simulink model "FIRB"  (R2020a)
settings: Solver=VariableStepAuto  StartTime=0.0  StopTime=300  RelTol=1e-3
InitFcn:
  | variableCalc
values from neighbouring files (symbols this model uses):
  aD1 = 10    [variableCalc.m]
  aD2 = 1    [variableCalc.m]
  Alin = [(-1),0,0,0;1,0,0,0;(-1),0,0,0.981E1;0,0,1,0]    [Matrix.m]
  bd = zeros(3,1)    [variableCalc.m]
  Blin = [1;0;1;0]    [Matrix.m]
  cAll = eye(length(Alin))    [variableCalc.m]
  cd = eye(3)    [variableCalc.m]
  d0 = [aD1;0;aD2]    [variableCalc.m]
  dAll = zeros(length(Alin),1)    [variableCalc.m]
  dd = zeros(3,1)    [variableCalc.m]
  S = [0 0 0 ... (first row only)    [variableCalc.m]
  wD1 = 10    [variableCalc.m]
  wD2 = 0.1    [variableCalc.m]
  x0 = [0;1;0;1]    [variableCalc.m]
settings Model: Creator=alfystar  LastModifiedBy=alfystar

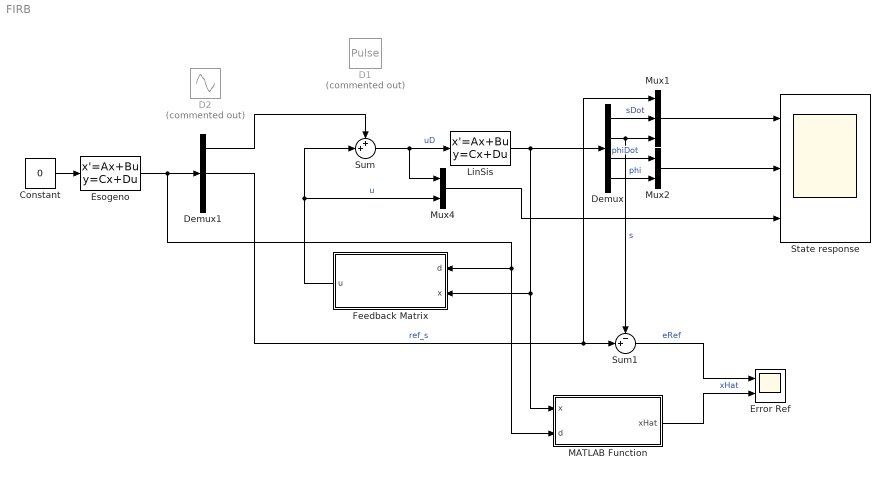
== system FIRB ==
  Constant : Constant  Value=0
  D1 : DiscretePulseGenerator  Commented=on  PulseType=Time based  Amplitude=aD1  Period=wD1  PulseWidth=50
  D2 : Sin  Commented=on  Amplitude=aD2  Frequency=wD2  SampleTime=0
  Demux : Demux
  Demux1 : Demux  Outputs=3
  Error Ref : Scope  NumInputPorts=2
  Esogeno : StateSpace  A=S  B=bd  C=cd  D=dd  InitialCondition=d0
  Feedback Matrix : MATLAB Function  TreatAsAtomicUnit=on
  LinSis : StateSpace  A=Alin  B=Blin  C=cAll  D=dAll  InitialCondition=x0
  MATLAB Function : MATLAB Function  TreatAsAtomicUnit=on
  Mux1 : Mux  Inputs=3
  Mux2 : Mux  Inputs=2
  Mux4 : Mux  Inputs=2
  State response : Scope  NumInputPorts=3
  Sum : Sum  Inputs=++|
  Sum1 : Sum  Inputs=-+|
  wires:
  LinSis/1 -> MATLAB Function/1(x), Feedback Matrix/2(x), Demux/1
  Demux/3 -> Mux2/1  "phiDot"
  Demux/4 -> Mux2/2  "phi"
  Mux1/1 -> State response/1
  Feedback Matrix/1(u) -> Sum/2, Mux4/2  "u"
  Demux/1 -> Mux1/2  "sDot"
  Demux/2 -> Mux1/3, Sum1/1  "s"
  Demux1/2 -> Sum1/2, Mux1/1  "ref_s"
  Mux2/1 -> State response/2
  Sum/1 -> Mux4/1, LinSis/1  "uD"
  Esogeno/1 -> Demux1/1, MATLAB Function/2(d), Feedback Matrix/1(d)
  Constant/1 -> Esogeno/1
  Mux4/1 -> State response/3
  Demux1/1 -> Sum/1
  Sum1/1 -> Error Ref/1  "eRef"
  MATLAB Function/1(xHat) -> Error Ref/2  "xHat"

== matlab function FIRB/MATLAB Function ==
  data: x input; xHat output; d input
function xHat = baseChange(x,d)

coder.extrinsic('evalin', 'assignin')
PiMat = zeros(4,3);                  % Needed in order to set variable class correctly
PiMat = evalin('base','PiMat'); % Read value from workspace


xHat = x-PiMat*d;
end

== matlab function FIRB/Feedback Matrix ==
  data: d input; x input; u output
function u = feedMatrix(d,x)

coder.extrinsic('evalin', 'assignin')
K = zeros(1,4);                  % Needed in order to set variable class correctly
K = evalin('base','K'); % Read value from workspace

L = zeros(1,3);                  % Needed in order to set variable class correctly
L = evalin('base','L'); % Read value from workspace

% x(2)=x(2)-d(2);

u=-K*x+L*d;
